simulink model "quadrant_map"  (Simulink 6.6)
settings: Solver=VariableStepDiscrete  StartTime=0.0  StopTime=6  RelTol=1e-3
StopFcn:
  | figure(2)
  | hold off
  | axis([-0.5 0.5 -0.5 0.5]);
  | plot([-0.5 0.5],[0 0],'k');
  | hold on
  | plot([0 0],[-0.5 0.5],'k','LineWidth',2);
  | markcolour = ['r' 'b' 'k' 'g' 'y' 'm' 'c'];
  | n = 14;
  | for i = 1:length(x_in)
  |    markcolour_index = 1+rem(i,length(markcolour));
  |    plot([0 x_out(i)],[0 y_out(i)],'k:', 'Color', markcolour(markcolour_index));
  |    plot(x_out(i),y_out(i),'k-o','MarkerFaceColor',markcolour(markcolour_index),'MarkerSize',15,'LineWidth',2);
  |    plot([0 x_in(i)],[0 y_in(i)],'k:', 'Color', markcolour(markcolour_index));
  |    plot(x_in(i),y_in(i),'k-s','MarkerFaceColor',markcolour(markcolour_index),'MarkerSize',10,'LineWidth',2);
  | end
  | xlabel('X');
  | ylabel('Y');
  | title('Squares: Inputs; Circles: Mapped Inputs');
  | axis equal
libraries: xbsIndex_r4 x13
settings Model: Creator=lcrockett  LastModifiedBy=lcrockett
settings DataIOCC: SignalLoggingName=sigsOut
settings OptimizationCC: InlineParams=on  InlineInvariantSignals=on
settings DebuggingCC: SignalResolutionControl=TryResolveAllWithWarning  SolverPrmCheckMsg=none  MultiTaskDSMMsg=warning  MultiTaskCondExecSysMsg=none  StrictBusMsg=None
settings HardwareCC: TargetUnknown=on
settings RTWCC: IncludeERTFirstTime=on
settings GRTTargetCC: ModelReferenceCompliant=off  MatFileLogging=off

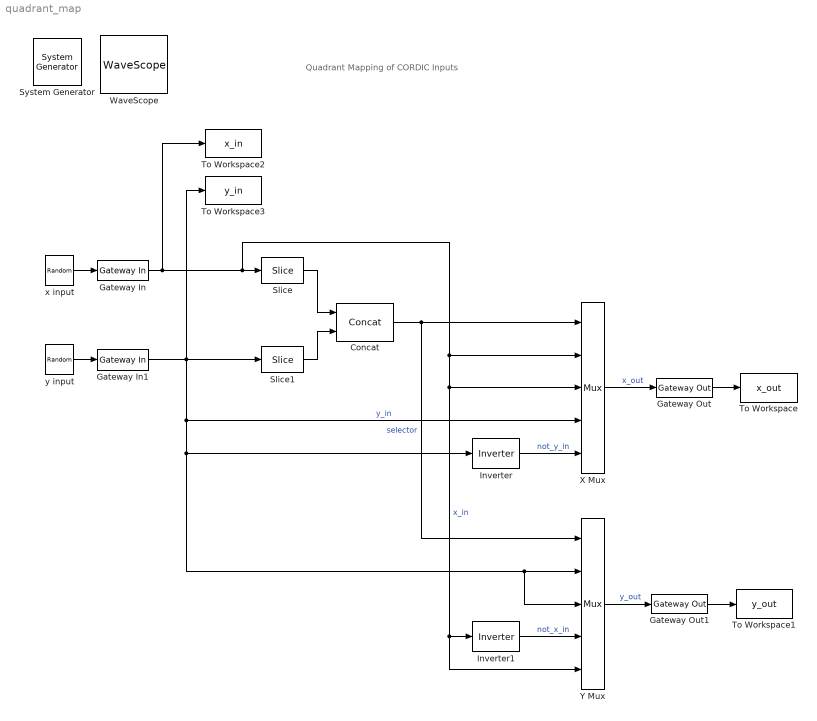
== system quadrant_map ==
  note: Quadrant Mapping of CORDIC Inputs
  " System Generator" : xbsIndex_r4/ System Generator  Tag=genX  SystemSampleTime=-1  xilinxfamily=virtex2p  part=xc2vp30  speed=-7  package=ff896  synthesis_tool=XST  clock_wrapper=Clock Enables  directory=./netlist  testbench=off  simulink_period=1  sysclk_period=100  dcm_input_clock_period=100  incr_netlist=off  trim_vbits=Everywhere in SubSystem  dbl_ovrd=According to Block Masks  core_generation=According to Block Masks  run_coregen=off  deprecated_control=off  eval_field=0  block_type=sysgen
      settings: block_version=9.2.01
  Concat : xbsIndex_r4/Concat  num_inputs=2  dbl_ovrd=off  block_type=concat
      settings: block_version=10.1.2
  Gateway In : xbsIndex_r4/Gateway In  arith_type="Signed  (2's comp)"  n_bits=16  bin_pt=14  quantization=Truncate  overflow=Wrap  period=1  dbl_ovrd=off  timing_constraint=None  locs_specified=off  LOCs={}  block_type=gatewayin
      settings: infoedit="Gateway in block.  Converts inputs of type Simulink integer, double and fixed point to  Xilinx fixed point type.<P><P>Hardware notes:  In hardware these blocks become top level input ports."  xl_area=[0, 0, 0, 0, 0, 0, 0]  block_version=VER_STRING_GOES_HERE
  Gateway In1 : xbsIndex_r4/Gateway In  arith_type="Signed  (2's comp)"  n_bits=16  bin_pt=14  quantization=Truncate  overflow=Wrap  period=1  dbl_ovrd=off  timing_constraint=None  locs_specified=off  LOCs={}  block_type=gatewayin
      settings: infoedit="Gateway in block.  Converts inputs of type Simulink integer, double and fixed point to  Xilinx fixed point type.<P><P>Hardware notes:  In hardware these blocks become top level input ports."  xl_area=[0, 0, 0, 0, 0, 0, 0]  block_version=VER_STRING_GOES_HERE
  Gateway Out : xbsIndex_r4/Gateway Out  hdl_port=on  timing_constraint=None  locs_specified=off  LOCs={}  block_type=gatewayout
      settings: infoedit="Gateway out block.  Converts Xilinx fixed point inputs into ouputs of type Simulink integer, double, or fixed point.<P><P>Hardware notes:  In hardware these blocks become top level output ports or are discarded, depending on how they are configured."  block_version=10.1
  Gateway Out1 : xbsIndex_r4/Gateway Out  hdl_port=on  timing_constraint=None  locs_specified=off  LOCs={}  block_type=gatewayout
      settings: infoedit="Gateway out block.  Converts Xilinx fixed point inputs into ouputs of type Simulink integer, double, or fixed point.<P><P>Hardware notes:  In hardware these blocks become top level output ports or are discarded, depending on how they are configured."  block_version=10.1
  Inverter : xbsIndex_r4/Inverter  en=off  latency=0  dbl_ovrd=off  block_type=inv
      settings: block_version=10.1.2
  Inverter1 : xbsIndex_r4/Inverter  en=off  latency=0  dbl_ovrd=off  block_type=inv
      settings: block_version=10.1.2
  Slice : xbsIndex_r4/Slice  nbits=1  boolean_output=on  mode=Upper Bit Location + Width  bit1=0  base1=MSB of Input  bit0=0  base0=LSB of Input  dbl_ovrd=off  block_type=slice
      settings: infoedit="Extracts a given range of bits from each input sample and presents it at the output.  The output type is ordinarily unsigned with binary point at zero, but can be Boolean when the slice is one bit wide.<P><P>Hardware notes: In hardware this block costs nothing."  block_version=VER_STRING_GOES_HERE
  Slice1 : xbsIndex_r4/Slice  nbits=1  boolean_output=on  mode=Upper Bit Location + Width  bit1=0  base1=MSB of Input  bit0=0  base0=LSB of Input  dbl_ovrd=off  block_type=slice
      settings: infoedit="Extracts a given range of bits from each input sample and presents it at the output.  The output type is ordinarily unsigned with binary point at zero, but can be Boolean when the slice is one bit wide.<P><P>Hardware notes: In hardware this block costs nothing."  block_version=VER_STRING_GOES_HERE
  To Workspace : ToWorkspace  VariableName=x_out  SampleTime=-1  SaveFormat=Array
  To Workspace1 : ToWorkspace  VariableName=y_out  SampleTime=-1  SaveFormat=Array
  To Workspace2 : ToWorkspace  VariableName=x_in  SampleTime=-1  SaveFormat=Array
  To Workspace3 : ToWorkspace  VariableName=y_in  SampleTime=-1  SaveFormat=Array
  WaveScope : xbsIndex_r4/WaveScope  block_type=wavescope
      settings: block_version=10.1.2
  X Mux : xbsIndex_r4/Mux  inputs=4  en=off  latency=0  precision=User Defined  arith_type="Signed  (2's comp)"  n_bits=16  bin_pt=14  quantization=Truncate  overflow=Wrap  dbl_ovrd=off  block_type=mux
      settings: xl_area=[0, 0, 0, 0, 0, 0, 0]  block_version=VER_STRING_GOES_HERE
  Y Mux : xbsIndex_r4/Mux  inputs=4  en=off  latency=0  precision=User Defined  arith_type="Signed  (2's comp)"  n_bits=16  bin_pt=14  quantization=Truncate  overflow=Wrap  dbl_ovrd=off  block_type=mux
      settings: xl_area=[0, 0, 0, 0, 0, 0, 0]  block_version=VER_STRING_GOES_HERE
  x input : UniformRandomNumber  Minimum=-0.5  Maximum=0.5  Seed=57  SampleTime=1
  y input : UniformRandomNumber  Minimum=-0.5  Maximum=0.5  Seed=9846  SampleTime=1
  wires:
  x input/1 -> Gateway In/1
  y input/1 -> Gateway In1/1
  Gateway In/1 -> To Workspace2/1, Slice/1, X Mux/2, X Mux/3, Y Mux/5, Inverter1/1  "x_in"
  Gateway In1/1 -> To Workspace3/1, Slice1/1, X Mux/4, Inverter/1, Y Mux/2, Y Mux/3  "y_in"
  Slice/1 -> Concat/1
  Gateway Out/1 -> To Workspace/1
  Gateway Out1/1 -> To Workspace1/1
  Slice1/1 -> Concat/2
  X Mux/1 -> Gateway Out/1  "x_out"
  Y Mux/1 -> Gateway Out1/1  "y_out"
  Concat/1 -> X Mux/1, Y Mux/1  "selector"
  Inverter/1 -> X Mux/5  "not_y_in"
  Inverter1/1 -> Y Mux/4  "not_x_in"
